simulink model "chap1_7"  (R2016a)
settings: Solver=ode45  StartTime=0.0  StopTime=1.0  FixedStep=0.001  RelTol=1e-3
undefined symbols (not defined in the file or in its folder): chap1_7f
settings Model: Creator=zhanghankui  LastModifiedBy=zhanghankui

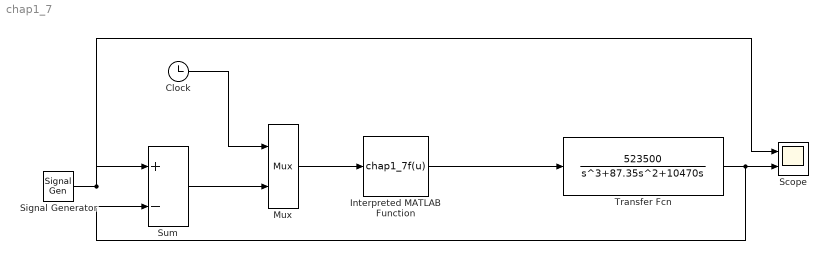
== system chap1_7 ==
  Clock : Clock
  Interpreted MATLAB Function : MATLABFcn  MATLABFcn=chap1_7f(u)
  Mux : Mux  Inputs=2
  Scope : Scope  NumInputPorts=2
  Signal Generator : SignalGenerator  Amplitude=0.05
  Sum : Sum  Inputs=|+-
  Transfer Fcn : TransferFcn  Numerator=[523500]  Denominator=[1 87.35 10470 0]
  wires:
  Signal Generator/1 -> Scope/1, Sum/1
  Sum/1 -> Mux/2
  Clock/1 -> Mux/1
  Transfer Fcn/1 -> Sum/2, Scope/2
  Mux/1 -> Interpreted MATLAB Function/1
  Interpreted MATLAB Function/1 -> Transfer Fcn/1
